simulink model "Problem2"  (R2020b)
settings: Solver=VariableStepAuto  StartTime=0.0  StopTime=100  RelTol=1e-3
model workspace (MAT data in the model file):
  Sig = Simulink.Signal
  Sig.DataType = 'auto'
  Sig.Dimensions = -1
  Sig.DimensionsMode = 'auto'
  Sig.Complexity = 'auto'
  Sig.SampleTime = -1
  Sig.SamplingMode = 'auto'
  b1 = 350
  k1 = 50000
  k2 = 50000
  m1 = 2500
  m2 = 320
  stin = [0 0 0 0 0 0 0 0 0 0 0 0 ... (1001 elements, 1001x1)]
  t = [0 0.01 0.02 0.03 0.04 0.05 0.06 0.07 0.08 0.09 0.1 0.11 ... (1001 elements, 1001x1)]
settings Model: ModifiedByFormat=Dell  OrderedModelArguments=off  Creator=Dell  LastModifiedBy=Dell
settings DataIOCC: ExternalInput=[t, stin]  LoadExternalInput=on

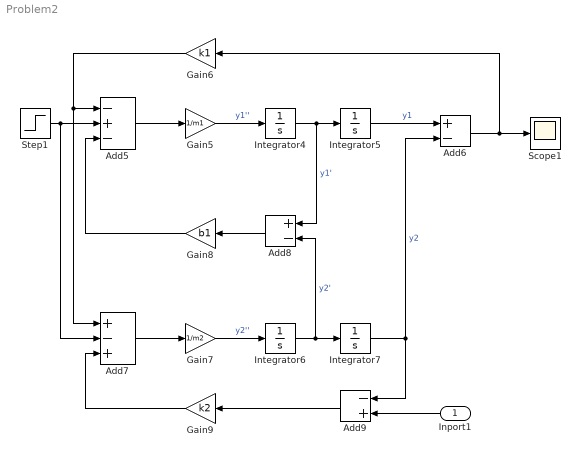
== system Problem2 ==
  Inport1 : Inport
  Add5 : Sum  Inputs=-+-
  Add6 : Sum  Inputs=+-
  Add7 : Sum  Inputs=+-+
  Add8 : Sum  Inputs=+-
  Add9 : Sum  Inputs=-+
  Gain5 : Gain  Gain=1/m1
  Gain6 : Gain  Gain=k1
  Gain7 : Gain  Gain=1/m2
  Gain8 : Gain  Gain=b1
  Gain9 : Gain  Gain=k2
  Integrator{4..7} (4 alike) : Integrator
  Scope1 : Scope
  Step1 : Step  SampleTime=0
  wires:
  Step1/1 -> Add7/2, Add5/2
  Add5/1 -> Gain5/1
  Gain5/1 -> Integrator4/1  "y1''"
  Integrator4/1 -> Add8/1, Integrator5/1  "y1'"
  Integrator5/1 -> Add6/1  "y1"
  Add6/1 -> Gain6/1, Scope1/1
  Gain6/1 -> Add7/1, Add5/1
  Add7/1 -> Gain7/1
  Gain7/1 -> Integrator6/1  "y2''"
  Integrator6/1 -> Add8/2, Integrator7/1  "y2'"
  Integrator7/1 -> Add9/1, Add6/2  "y2"
  Add8/1 -> Gain8/1
  Gain8/1 -> Add5/3
  Inport1/1 -> Add9/2
  Add9/1 -> Gain9/1
  Gain9/1 -> Add7/3
